simulink model "AKident"  (R2023b)
settings: Solver=ode45  StartTime=0.0  StopTime=tend  MaxStep=0.01  RelTol=1e-3  EnableMultiTasking=on
values from neighbouring files (symbols this model uses):
  sigma2v = 0    [Lab2_Z2_1_Gs.m]    (also in Lab2_Z2_1_Gz.m = wektor_var(j))
  Tp = 1    [Lab2_Z2_1_Gs.m]    (also in Lab2_Z2_1_Gz.m)
libraries: simulink x1
settings Model: Creator=Rafał  LastModifiedBy=Rafał
settings SolverCC: AlgebraicLoopSolver=TrustRegion
settings DataIOCC: LimitDataPoints=on  SaveFormat=Array  SignalLoggingSaveFormat=ModelDataLogs  ReturnWorkspaceOutputs=off
settings OptimizationCC: InitFltsAndDblsToZero=on  LifeSpan=inf
settings DebuggingCC: SaveWithParameterizedLinksMsg=none  UnderspecifiedInitializationDetection=Classic  MergeDetectMultiDrivingBlocksExec=none  SignalResolutionControl=TryResolveAllWithWarning  SolverPrmCheckMsg=warning  MultiTaskDSMMsg=warning  MultiTaskCondExecSysMsg=none  FcnCallInpInsideContextMsg=warning  UnconnectedInputMsg=warning  UnconnectedOutputMsg=warning  UnconnectedLineMsg=warning  SFUnexpectedBacktrackingDiag=warning  SFNoUnconditionalDefaultTransitionDiag=warning  SFExecutionAtInitializationDiag=none  ArithmeticOperatorsInVariantConditions=warning
settings HardwareCC: ProdBitPerPointer=32  ProdBitPerSizeT=32  ProdBitPerPtrDiffT=32  ProdLargestAtomicFloat=None  ProdIntDivRoundTo=Undefined  ProdEndianess=Unspecified  ProdWordSize=32  ProdHWDeviceType=32-bit Generic
settings ModelReferenceCC: PropagateSignalLabelsOutOfModel=off
settings CodeAppCC: StateflowObjectComments=on
settings GRTTargetCC: TargetFcnLib=ansi_tfl_tmw.mat  TargetLangStandard=C89/C90 (ANSI)  CombineOutputUpdateFcns=off  GRTInterface=on
settings ConfigComp: CovMetricSettings=dw  CovSaveCumulativeToWorkspaceVar=on  CovSaveSingleToWorkspaceVar=on

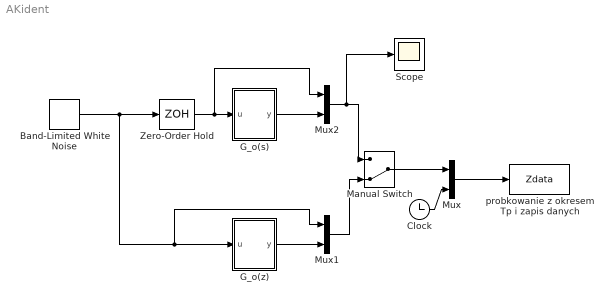
== system AKident ==
  Band-Limited White Noise : simulink/Sources/Band-Limited White Noise  Cov=[0.5]*Tp  Ts=Tp  seed=[23341]
  Clock : Clock
  G_o(s) : Subsystem
  G_o(z) : Subsystem
  Manual Switch : ManualSwitch  CurrentSetting=0
  Mux : Mux  Inputs=2
  Mux1 : Mux  Inputs=2
  Mux2 : Mux  Inputs=2
  Scope : Scope
  Zero-Order Hold : ZeroOrderHold  SampleTime=Tp
  probkowanie z okresem Tp i zapis danych : ToWorkspace  VariableName=Zdata  SampleTime=Tp
  wires:
  Zero-Order Hold/1 -> G_o(s)/1(u), Mux2/1
  Band-Limited White Noise/1 -> Zero-Order Hold/1, G_o(z)/1(u), Mux1/1
  Mux/1 -> probkowanie z okresem Tp i zapis danych/1
  Manual Switch/1 -> Mux/1
  Clock/1 -> Mux/2
  Mux1/1 -> Manual Switch/2
  Mux2/1 -> Scope/1, Manual Switch/1
  G_o(s)/1(y) -> Mux2/2
  G_o(z)/1(y) -> Mux1/2

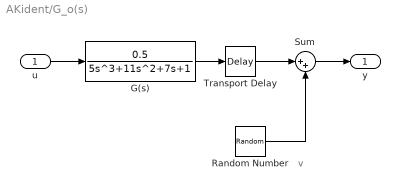
== system AKident/G_o(s) ==
  note: v
  u : Inport
  G(s) : TransferFcn  Numerator=[0.5]  Denominator=[5 11 7 1]
  Random Number : RandomNumber  Variance=sigma2v  Seed=159  SampleTime=Tp*0.1
  Sum : Sum  Inputs=|++
  Transport Delay : TransportDelay  DelayTime=3
  y : Outport
  wires:
  G(s)/1 -> Transport Delay/1
  u/1 -> G(s)/1
  Random Number/1 -> Sum/2
  Sum/1 -> y/1
  Transport Delay/1 -> Sum/1

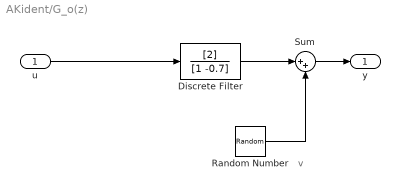
== system AKident/G_o(z) ==
  note: v
  u : Inport
  Discrete Filter : DiscreteFilter  Numerator=[2]  Denominator=[1 -0.7]  SampleTime=Tp
  Random Number : RandomNumber  Variance=sigma2v  Seed=159  SampleTime=Tp
  Sum : Sum  Inputs=|++
  y : Outport
  wires:
  u/1 -> Discrete Filter/1
  Random Number/1 -> Sum/2
  Sum/1 -> y/1
  Discrete Filter/1 -> Sum/1
